simulink model "iC_3ph_MR2"  (Simulink 7.9)
settings: Solver=ode14x  StartTime=0.0  StopTime=20/60  FixedStep=Ts1  RelTol=1e-3
PostLoadFcn:
  | , if any(exist('dsrtsu_mdlpostloadfcn', 'file') == [2, 3, 6]), try dsrtsu_mdlpostloadfcn('Execute', bdroot); catch fprintf('Error in PostLoadFcn (dsrtsu_mdlpostloadfcn) for model "%s":\n %s\n', bdroot, lasterr); end, end,
InitFcn:
  | iC_ini
values from neighbouring files (symbols this model uses):
  C = Cideal+deltaC    (= 4e-05)    [IMC_calculo_limites_thetas.m]    (also in IMC_ini.m; JORGE_controlador_LCL_malha_interna.m; LCL_PAPM.m; R_in_LCL.m)
  excitacao_persistente = 0    [iC_ini.m]    (also in vC_ini.m)
  flag_time = 60/60    (= 1)    [iC_ini.m]    (also in vC_ini.m = 0)
  init_time = 60/60    (= 1)    [iC_ini.m]    (also in vC_ini.m)
  L1 = L1ideal+deltaL1    (= 0.002)    [IMC_calculo_limites_thetas.m]    (also in IMC_ini.m; LCL_PAPM.m; R_in_LCL.m; calculo_FTs.m)
  L2 = L2ideal+deltaL2+Lgideal+deltaLg    (= 0.002)    [IMC_calculo_limites_thetas.m]    (also in IMC_ini.m; LCL_PAPM.m; R_in_LCL.m; calculo_FTs.m)
  param_change_time = 60/60    (= 1)    [iC_ini.m]    (also in vC_ini.m)
  R1 = R1ideal+deltaR1    (= 1)    [IMC_calculo_limites_thetas.m]    (also in IMC_ini.m; R_in_LCL.m = 0; gera_resultados.m = 0; iC_ini.m = 0)
  R2 = R2ideal+deltaR2+Rgideal+deltaRg    (= 1)    [IMC_calculo_limites_thetas.m]    (also in IMC_ini.m; R_in_LCL.m = 0; gera_resultados.m = 0; iC_ini.m = 0)
  R_init = 10    [iC_ini.m]    (also in vC_ini.m)
  ref_phaseInv_time = 60/60    (= 1)    [iC_ini.m]    (also in vC_ini.m)
  ref_step_time = 60/60    (= 1)    [iC_ini.m]    (also in vC_ini.m)
  short_OFF_time = 61/60    (= 1.01666666667)    [iC_ini.m]    (also in vC_ini.m)
  short_ON_time = 60/60    (= 1)    [iC_ini.m]    (also in vC_ini.m)
  Ts = 0.5    [IMC_calculo_limites_thetas.m]    (also in IMC_datta_ini.m; IMC_ini.m = 8.33333333333e-05; JORGE_controlador_LCL_malha_interna.m = 8.33333333333e-05; LCL_PAPM.m = 8.33333333333e-05)
  Ts1 = Ts/10    (= 8.33333333333e-06)    [iC_ini.m]    (also in vC_ini.m)
  VCC = 1700    [iC_ini.m]    (also in vC_ini.m = 1200)
undefined symbols (not defined in the file or in its folder): D1, Delta
libraries: powerlib x38, powerlib_extras x1
(part 2 of 3)

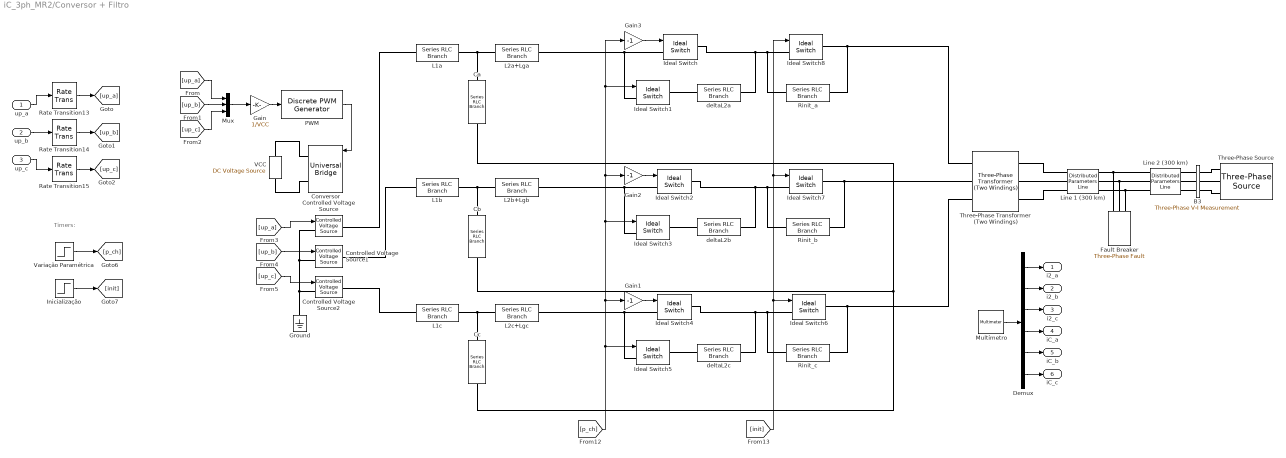
== system iC_3ph_MR2/Conversor + Filtro ==
  note: Timers:
  up_a : Inport
  up_b : Inport  Port=2
  up_c : Inport  Port=3
  B3 : powerlib/Measurements/Three-Phase V-I Measurement  VoltageMeasurement=no  SetLabelV=on  LabelV=Vabc_B3  Vpu=on  VpuLL=off  CurrentMeasurement=no  SetLabelI=on  LabelI=Iabc_B3  Ipu=on  Pbase=100e6  Vbase=735e3  OutputType=Complex  PhasorSimulation=off  PSBequivalent=0
  Ca : powerlib/Elements/Series RLC Branch  LConnTagsString=__new0  RConnTagsString=__new0  BranchType=C  Resistance=1  Inductance=1e-3  SetiL0=off  InitialCurrent=0  Capacitance=C  Setx0=off  InitialVoltage=0  Measurements=Branch current
  Cb : powerlib/Elements/Series RLC Branch  LConnTagsString=__new0  RConnTagsString=__new0  BranchType=C  Resistance=1  Inductance=1e-3  SetiL0=off  InitialCurrent=0  Capacitance=C  Setx0=off  InitialVoltage=0  Measurements=Branch current
  Cc : powerlib/Elements/Series RLC Branch  LConnTagsString=__new0  RConnTagsString=__new0  BranchType=C  Resistance=1  Inductance=1e-3  SetiL0=off  InitialCurrent=0  Capacitance=C  Setx0=off  InitialVoltage=0  Measurements=Branch current
  Controlled Voltage Source : powerlib/Electrical Sources/Controlled Voltage Source  Initialize=on  Source_Type=AC  Amplitude=0  Phase=0  Frequency=0  Measurements=None
  Controlled Voltage Source1 : powerlib/Electrical Sources/Controlled Voltage Source  Initialize=on  Source_Type=AC  Amplitude=0  Phase=0  Frequency=0  Measurements=None
  Controlled Voltage Source2 : powerlib/Electrical Sources/Controlled Voltage Source  Initialize=on  Source_Type=AC  Amplitude=0  Phase=0  Frequency=0  Measurements=None
  Conversor : powerlib/Power Electronics/Universal Bridge  Arms=3  SnubberResistance=1e5  SnubberCapacitance=inf  Device=IGBT / Diodes  Ron=1e-3  Lon=0  ForwardVoltages="[  0  0  ]"  ForwardVoltage=0  GTOparameters=[ 10e-6 , 20e-6 ]  IGBTparameters=[ 1e-6 , 2e-6 ]  Measurements=UAB UBC UCA UDC voltages  Measurements_2=None  converterType=Rectifier
  Demux : Demux  Outputs=6
  Fault Breaker : powerlib/Elements/Three-Phase Fault  FaultA=on  FaultB=off  FaultC=off  FaultResistance=0.001  GroundFault=on  GroundResistance=1  External=off  SwitchStatus=[1 0]  SwitchTimes=[ short_ON_time short_OFF_time ]  InitialStates=[0 0 1]  SnubberResistance=inf  SnubberCapacitance=inf  Measurements=Fault currents
  Gain : Gain  Gain=1/VCC  SampleTime=Ts1
  Gain1 : Gain  Gain=-1  SampleTime=Ts1
  Gain2 : Gain  Gain=-1  SampleTime=Ts1
  Gain3 : Gain  Gain=-1  SampleTime=Ts1
  Ground : powerlib/Elements/Ground  LConnTagsString=a
  Ideal Switch : powerlib/Power Electronics/Ideal Switch  Ron=0.001  Lon=0  IC=1  Rs=1e5  Cs=inf  Measurements=off
  Ideal Switch{1,3,5..8} (6 alike) : powerlib/Power Electronics/Ideal Switch  Ron=0.001  Lon=0  IC=0  Rs=1e5  Cs=inf  Measurements=off
  Ideal Switch2 : powerlib/Power Electronics/Ideal Switch  Ron=0.001  Lon=0  IC=1  Rs=1e5  Cs=inf  Measurements=off
  Ideal Switch4 : powerlib/Power Electronics/Ideal Switch  Ron=0.001  Lon=0  IC=1  Rs=1e5  Cs=inf  Measurements=off
  Inicialização : Step  Time=init_time  SampleTime=Ts1
  L1a : powerlib/Elements/Series RLC Branch  LConnTagsString=__new0  RConnTagsString=__new0  BranchType=RL  Resistance=R1  Inductance=L1  SetiL0=off  InitialCurrent=0  Capacitance=1e-6  Setx0=off  InitialVoltage=0  Measurements=Branch current
  L1b : powerlib/Elements/Series RLC Branch  LConnTagsString=__new0  RConnTagsString=__new0  BranchType=RL  Resistance=R1  Inductance=L1  SetiL0=off  InitialCurrent=0  Capacitance=1e-6  Setx0=off  InitialVoltage=0  Measurements=None
  L1c : powerlib/Elements/Series RLC Branch  LConnTagsString=__new0  RConnTagsString=__new0  BranchType=RL  Resistance=R1  Inductance=L1  SetiL0=off  InitialCurrent=0  Capacitance=1e-6  Setx0=off  InitialVoltage=0  Measurements=None
  L2a+Lga : powerlib/Elements/Series RLC Branch  LConnTagsString=__new0  RConnTagsString=__new0  BranchType=RL  Resistance=R2  Inductance=L2  SetiL0=off  InitialCurrent=0  Capacitance=1e-6  Setx0=off  InitialVoltage=0  Measurements=Branch current
  L2b+Lgb : powerlib/Elements/Series RLC Branch  LConnTagsString=__new0  RConnTagsString=__new0  BranchType=RL  Resistance=R2  Inductance=L2  SetiL0=off  InitialCurrent=0  Capacitance=1e-6  Setx0=off  InitialVoltage=0  Measurements=Branch current
  L2c+Lgc : powerlib/Elements/Series RLC Branch  LConnTagsString=__new0  RConnTagsString=__new0  BranchType=RL  Resistance=R2  Inductance=L2  SetiL0=off  InitialCurrent=0  Capacitance=1e-6  Setx0=off  InitialVoltage=0  Measurements=Branch current
  Line 1 (300 km) : powerlib/Elements/Distributed Parameters Line  Phases=3  Frequency=60  Resistance=[0.01273 0.3864]  Inductance="[0.9337e-3  4.1264e-3]"  Capacitance=[12.74e-9 7.751e-9]  Length=300  x1=[-0.0017 -2.07986760325051e-10 -7396.02996094136 -52768.9690973412;-0.00169166666666667 -2.08294895140375e-10 -7230.21513006747 -52791.9439683011;-0.00168333333333333 -2.08600974169177e-10 -7064.32893988922 -52814.3978040869;-0.001675 -2.08904994390579e-10 -6898.37302763631 -52836.3303830884;-0.00166666666666667 -2.09206952804025e-10 -6732.3490312266 -52857.74148884;-0.00165833333333333 -2.09506846429307e-10 -6566.25858924991 -52878.6309100226;-0.00165 -2.09804672306596e-10 -6400.10334095186 -52898.9984404661;-0.00164166666666667 -2.10100427496471e-10 -6233.88492621764 -52918.8438791511;-0.00163333333333333 -2.10394109079948e-10 -6067.60498555594 -52938.1670302113;-0.001625 -2.10685714158508e-10 -5901.26516008262 -52956.9677029349;-0.00161666666666667 -2.10975239854126e-10 -5734.86709150461 -52975.2457117668;-0.00160833333333333 -2.112626833093e-10 -5568.41242210365 -52993.0008763106;-0.0016 -2.11548041687081e-10 -5401.90279472016 -53010.2330213298;-0.00159166666666667 -2.11831312171096e-10 -5235.33985273692 -53026.9419767503;-0.00158333333333333 -2.12112491965579e-10 -5068.72524006292 -53043.1275776612;-0.001575 -2.123915782954e-10 -4902.06060111712 -53058.7896643173;-0.00156666666666667 -2.12668568406089e-10 -4735.34758081225 -53073.9280821402;-0.00155833333333333 -2.12943459563866e-10 -4568.58782453848 -53088.5426817197;-0.00155 -2.13216249055666e-10 -4401.7829781473 -53102.6333188156;-0.00154166666666667 -2.13486934189166e-10 -4234.9346879352 -53116.1998543591;-0.00153333333333333 -2.13755512292814e-10 -4068.04460062744 -53129.2421544539;-0.001525 -2.14021980715852e-10 -3901.11436336179 -53141.7600903777;-0.00151666666666667 -2.14286336828345e-10 -3734.14562367234 -53153.7535385837;-0.00150833333333333 -2.14548578021204e-10 -3567.14002947312 -53165.2223807013;-0.0015 -2.14808701706215e-10 -3400.09922904191 -53176.1665035377;-0.00149166666666667 -2.15066705316062e-10 -3233.02487100399 -53186.5857990787;-0.00148333333333333 -2.15322586304353e-10 -3065.91860431582 -53196.4801644902;-0.001475 -2.15576342145647e-10 -2898.78207824879 -53205.8495021188;-0.00146666666666667 -2.15827970335475e-10 -2731.61694237293 -53214.6937194929;-0.00145833333333333 -2.16077468390369e-10 -2564.42484654063 -53223.0127293236;-0.00145 -2.16324833847885e-10 -2397.20744087041 -53230.8064495056;-0.00144166666666667 -2.16570064266624e-10 -2229.96637573055 -53238.0748031181;-0.00143333333333333 -2.16813157226262e-10 -2062.70330172282 -53244.8177184255;-0.001425 -2.17054110327569e-10 -1895.41986966626 -53251.0351288777;-0.00141666666666667 -2.17292921192435e-10 -1728.11773058079 -53256.7269731115;-0.00140833333333333 -2.17529587463894e-10 -1560.798535671 -53261.8931949507;-0.0014 -2.17764106806145e-10 -1393.46393630977 -53266.5337434068;-0.00139166666666667 -2.17996476904577e-10 -1226.11558402205 -53270.6485726794;-0.00138333333333333 -2.1822669546579e-10 -1058.75513046853 -53274.2376421568;-0.001375 -2.18454760217621e-10 -891.384227429309 -53277.3009164164;-0.00136666666666667 -2.18680668909162e-10 -724.004526787619 -53279.8383652248;-0.00135833333333333 -2.18904419310786e-10 -556.617680513551 -53281.8499635385;-0.00135 -2.19126009214166e-10 -389.225340647688 -53283.3356915038;-0.00134166666666667 -2.19345436432301e-10 -221.829159284855 -53284.2955344572;-0.00133333333333333 -2.19562698799531e-10 -54.4307885577764 -53284.7294829255;-0.001325 -2.19777794171565e-10 112.968119379217 -53284.6375326256;-0.00131666666666667 -2.19990720425499e-10 280.365912366477 -53284.0196844652;-0.00130833333333333 -2.20201475459835e-10 447.760938255375 -53282.8759445421;-0.0013 -2.20410057194508e-10 615.151544924574 -53281.2063241446;-0.00129166666666667 -2.206164635709e-10 782.536080296377 -53279.0108397512;-0.00128333333333333 -2.20820692551862e-10 949.912892352986 -53276.2895130304;-0.001275 -2.21022742121738e-10 1117.28032915284 -53273.0423708406;-0.00126666666666667 -2.2122261028638e-10 1284.63673884692 -53269.2694452298;-0.00125833333333333 -2.21420295073169e-10 ...(+11171 chars)]  x2=[-0.0017 -1.41909241010387e-10 -6618.00740677681 -48900.0765944437;-0.00169166666666667 -1.41941661559306e-10 -6464.3508795585 -48920.6263316871;-0.00168333333333333 -1.4197268120133e-10 -6310.63055180677 -48940.6932420988;-0.001675 -1.42002299630307e-10 -6156.8479406792 -48960.2771276263;-0.00166666666666667 -1.42030516553915e-10 -6003.00456394808 -48979.3777949846;-0.00165833333333333 -1.42057331693664e-10 -5849.10193998542 -48997.9950556578;-0.00165 -1.42082744784901e-10 -5695.141587748 -49016.1287259012;-0.00164166666666667 -1.42106755576808e-10 -5541.12502676231 -49033.7786267426;-0.00163333333333333 -1.42129363832408e-10 -5387.05377710966 -49050.9445839847;-0.001625 -1.42150569328568e-10 -5232.92935941108 -49067.6264282065;-0.00161666666666667 -1.42170371855996e-10 -5078.75329481233 -49083.8239947647;-0.00160833333333333 -1.42188771219251e-10 -4924.52710496894 -49099.5371237962;-0.0016 -1.42205767236737e-10 -4770.25231203114 -49114.7656602184;-0.00159166666666667 -1.42221359740712e-10 -4615.93043862884 -49129.5094537321;-0.00158333333333333 -1.42235548577283e-10 -4461.56300785664 -49143.7683588218;-0.001575 -1.42248333606413e-10 -4307.15154325876 -49157.542234758;-0.00156666666666667 -1.42259714701918e-10 -4152.69756881402 -49170.830945598;-0.00155833333333333 -1.42269691751471e-10 -3998.20260892078 -49183.6343601876;-0.00155 -1.42278264656604e-10 -3843.66818838194 -49195.9523521624;-0.00154166666666667 -1.42285433332704e-10 -3689.09583238982 -49207.7847999486;-0.00153333333333333 -1.4229119770902e-10 -3534.48706651119 -49219.1315867649;-0.001525 -1.4229555772866e-10 -3379.84341667214 -49229.9926006229;-0.00151666666666667 -1.42298513348593e-10 -3225.16640914306 -49240.367734329;-0.00150833333333333 -1.42300064539646e-10 -3070.45757052359 -49250.2568854846;-0.0015 -1.42300211286512e-10 -2915.71842772749 -49259.6599564879;-0.00149166666666667 -1.42298953587741e-10 -2760.95050796762 -49268.5768545344;-0.00148333333333333 -1.42296291455747e-10 -2606.15533874088 -49277.0074916179;-0.001475 -1.42292224916804e-10 -2451.3344478131 -49284.9517845313;-0.00146666666666667 -1.42286754011046e-10 -2296.48936320396 -49292.4096548678;-0.00145833333333333 -1.42279878792469e-10 -2141.62161317193 -49299.3810290211;-0.00145 -1.4227159932893e-10 -1986.7327261992 -49305.8658381866;-0.00144166666666667 -1.42261915702142e-10 -1831.82423097653 -49311.8640183619;-0.00143333333333333 -1.42250828007681e-10 -1676.89765638823 -49317.3755103474;-0.001425 -1.42238336354975e-10 -1521.95453149706 -49322.4002597467;-0.00141666666666667 -1.42224440867314e-10 -1366.99638552911 -49326.9382169678;-0.00140833333333333 -1.4220914168184e-10 -1212.0247478587 -49330.9893372228;-0.0014 -1.42192438949549e-10 -1057.04114799335 -49334.5535805287;-0.00139166666666667 -1.42174332835291e-10 -902.047115558609 -49337.630911708;-0.00138333333333333 -1.42154823517767e-10 -747.044180283017 -49340.2213003885;-0.001375 -1.42133911189524e-10 -592.03387198296 -49342.3247210043;-0.00136666666666667 -1.4211159605696e-10 -437.017720547588 -49343.9411527954;-0.00135833333333333 -1.42087878340316e-10 -281.997255923754 -49345.0705798083;-0.00135 -1.42062758273676e-10 -126.974008100849 -49345.7129908959;-0.00134166666666667 -1.42036236104964e-10 28.0504929042545 -49345.868379718;-0.00133333333333333 -1.42008312095944e-10 183.074717062311 -49345.536744741;-0.001325 -1.41978986522216e-10 338.09713434683 -49344.7180892378;-0.00131666666666667 -1.41948259673209e-10 493.116214749123 -49343.4124212884;-0.00130833333333333 -1.41916131852186e-10 648.130428293458 -49341.6197537792;-0.0013 -1.41882603376236e-10 803.138245052127 -49339.3401044029;-0.00129166666666667 -1.41847674576271e-10 958.138135160556 -49336.573495659;-0.00128333333333333 -1.41811345797024e-10 1113.12856883241 -49333.3199548526;-0.001275 -1.41773617397045e-10 1268.10801637467 -49329.5795140949;-0.00126666666666667 -1.41734489748699e-10 1423.07494820278 -49325.3522103026;-0.00125833333333333 -1.4169396323816e-10 ...(+11177 chars)]  x3=[-0.0017 -3.70381053816407e-13 -27.7294039862372 -193.67611553396;-0.00169166666666667 -3.70681312258177e-13 -27.1208166863507 -193.762274129979;-0.00168333333333333 -3.70977912225046e-13 -26.5119617149526 -193.846520370577;-0.001675 -3.71270850789691e-13 -25.9028450811956 -193.928853424279;-0.00166666666666667 -3.71560125060927e-13 -25.2934727968152 -194.009272478489;-0.00165833333333333 -3.71845732183734e-13 -24.6838508760696 -194.087776739504;-0.00165 -3.72127669339284e-13 -24.0739853356812 -194.16436543252;-0.00164166666666667 -3.72405933744971e-13 -23.4638821947765 -194.239037801636;-0.00163333333333333 -3.72680522654439e-13 -22.8535474748273 -194.311793109866;-0.001625 -3.72951433357606e-13 -22.2429871995909 -194.382630639146;-0.00161666666666667 -3.73218663180692e-13 -21.6322073950507 -194.451549690336;-0.00160833333333333 -3.73482209486246e-13 -21.0212140893568 -194.518549583234;-0.0016 -3.73742069673174e-13 -20.4100133127665 -194.583629656578;-0.00159166666666667 -3.73998241176761e-13 -19.7986110975845 -194.646789268054;-0.00158333333333333 -3.74250721468695e-13 -19.1870134781041 -194.708027794302;-0.001575 -3.74499508057101e-13 -18.5752264905468 -194.767344630923;-0.00156666666666667 -3.74744598486553e-13 -17.9632561730031 -194.824739192482;-0.00155833333333333 -3.74985990338108e-13 -17.351108565373 -194.88021091252;-0.00155 -3.75223681229327e-13 -16.7387897093064 -194.933759243553;-0.00154166666666667 -3.75457668814297e-13 -16.126305648143 -194.985383657079;-0.00153333333333333 -3.75687950783653e-13 -15.5136624268534 -195.035083643588;-0.001525 -3.75914524864606e-13 -14.9008660919787 -195.08285871256;-0.00151666666666667 -3.76137388820962e-13 -14.2879226915714 -195.128708392475;-0.00150833333333333 -3.76356540453143e-13 -13.6748382751354 -195.172632230814;-0.0015 -3.76571977598211e-13 -13.0616188935664 -195.214629794068;-0.00149166666666667 -3.76783698129889e-13 -12.4482705990921 -195.254700667737;-0.00148333333333333 -3.76991699958579e-13 -11.8347994452125 -195.292844456338;-0.001475 -3.77195981031389e-13 -11.2212114866404 -195.329060783407;-0.00146666666666667 -3.77396539332146e-13 -10.607512779241 -195.363349291503;-0.00145833333333333 -3.77593372881421e-13 -9.99370937997291 -195.395709642214;-0.00145 -3.77786479736546e-13 -9.3798073468279 -195.426141516155;-0.00144166666666667 -3.77975857991635e-13 -8.76581273877116 -195.454644612975;-0.00143333333333333 -3.78161505777601e-13 -8.15173161568156 -195.481218651362;-0.001425 -3.78343421262174e-13 -7.53757003829192 -195.50586336904;-0.00141666666666667 -3.78521602649923e-13 -6.92333406812905 -195.528578522775;-0.00140833333333333 -3.7869604818227e-13 -6.30902976745399 -195.549363888378;-0.0014 -3.78866756137506e-13 -5.69466319920217 -195.568219260705;-0.00139166666666667 -3.79033724830814e-13 -5.08024042692358 -195.585144453663;-0.00138333333333333 -3.7919695261428e-13 -4.46576751472298 -195.600139300206;-0.001375 -3.79356437876912e-13 -3.85125052719994 -195.613203652342;-0.00136666666666667 -3.79512179044655e-13 -3.23669552938895 -195.624337381129;-0.00135833333333333 -3.79664174580405e-13 -2.62210858669984 -195.633540376683;-0.00135 -3.79812422984029e-13 -2.00749576485755 -195.640812548174;-0.00134166666666667 -3.79956922792375e-13 -1.39286312984251 -195.646153823829;-0.00133333333333333 -3.80097672579287e-13 -0.778216747830726 -195.649564150931;-0.001325 -3.80234670955623e-13 -0.163562685133797 -195.651043495821;-0.00131666666666667 -3.80367916569263e-13 0.45109299186079 -195.6505918439;-0.00130833333333333 -3.80497408105128e-13 1.06574421674968 -195.648209199625;-0.0013 -3.80623144285187e-13 1.68038492317338 -195.643895586511;-0.00129166666666667 -3.80745123868477e-13 2.29500904487631 -195.637651047133;-0.00128333333333333 -3.80863345651106e-13 2.90961051576649 -195.62947564312;-0.001275 -3.80977808466275e-13 3.52418326997552 -195.619369455162;-0.00126666666666667 -3.81088511184281e-13 4.13872124191849 -195.607332583003;-0.00125833333333333 -3.81195452712534e-13 ...(+11162 chars)]  x4=[-0.0017 -8.97577288364198e-15 -97.1520132574431 -167.719905551199;-0.00169166666666667 -9.90341611680488e-15 -96.624627075456 -168.024289436398;-0.00168333333333333 -1.08309616072489e-14 -96.0962872474087 -168.327014989695;-0.001675 -1.17584002004744e-14 -95.5669989878018 -168.62807922331;-0.00166666666666667 -1.26857227430371e-14 -95.036767520497 -168.927479165861;-0.00165833333333333 -1.36129200826377e-14 -94.5055980786645 -169.225211862392;-0.00165 -1.45399830682128e-14 -93.9734959047326 -169.5212743744;-0.00164166666666667 -1.54669025500252e-14 -93.4404662503346 -169.815663779869;-0.00163333333333333 -1.63936693797535e-14 -92.9065143762582 -170.108377173294;-0.001625 -1.73202744105835e-14 -92.3716455523928 -170.399411665711;-0.00161666666666667 -1.82467084972975e-14 -91.8358650576778 -170.688764384729;-0.00160833333333333 -1.91729624963652e-14 -91.2991781800502 -170.976432474552;-0.0016 -2.00990272660334e-14 -90.761590216393 -171.262413096012;-0.00159166666666667 -2.10248936664168e-14 -90.2231064724823 -171.546703426596;-0.00158333333333333 -2.19505525595879e-14 -89.6837322629353 -171.829300660474;-0.001575 -2.2875994809667e-14 -89.1434729111575 -172.110202008525;-0.00156666666666667 -2.38012112829127e-14 -88.6023337492909 -172.389404698365;-0.00155833333333333 -2.4726192847812e-14 -88.0603201181603 -172.666905974378;-0.00155 -2.56509303751702e-14 -87.5174373672216 -172.942703097737;-0.00154166666666667 -2.65754147382014e-14 -86.9736908545083 -173.216793346436;-0.00153333333333333 -2.7499636812618e-14 -86.4290859465789 -173.489174015315;-0.001525 -2.84235874767214e-14 -85.8836280184641 -173.759842416088;-0.00151666666666667 -2.93472576114914e-14 -85.3373224536133 -174.028795877365;-0.00150833333333333 -3.02706381006767e-14 -84.7901746438421 -174.296031744685;-0.0015 -3.11937198308847e-14 -84.2421899892782 -174.561547380538;-0.00149166666666667 -3.21164936916715e-14 -83.6933738983091 -174.825340164392;-0.00148333333333333 -3.30389505756314e-14 -83.1437317875281 -175.087407492718;-0.001475 -3.39610813784875e-14 -82.5932690816807 -175.347746779018;-0.00146666666666667 -3.48828769991811e-14 -82.0419912136118 -175.606355453848;-0.00145833333333333 -3.58043283399615e-14 -81.4899036242113 -175.863230964844;-0.00145 -3.67254263064759e-14 -80.9370117623608 -176.11837077675;-0.00144166666666667 -3.76461618078593e-14 -80.3833210848798 -176.371772371439;-0.00143333333333333 -3.85665257568241e-14 -79.8288370564718 -176.623433247938;-0.001425 -3.94865090697496e-14 -79.2735651496702 -176.873350922457;-0.00141666666666667 -4.04061026667719e-14 -78.7175108447846 -177.121522928408;-0.00140833333333333 -4.13252974718735e-14 -78.1606796298466 -177.367946816436;-0.0014 -4.22440844129728e-14 -77.6030770005553 -177.612620154434;-0.00139166666666667 -4.31624544220135e-14 -77.0447084602237 -177.855540527577;-0.00138333333333333 -4.40803984350545e-14 -76.4855795197238 -178.096705538338;-0.001375 -4.49979073923588e-14 -75.9256956974325 -178.336112806516;-0.00136666666666667 -4.59149722384837e-14 -75.365062519177 -178.573759969257;-0.00135833333333333 -4.68315839223691e-14 -74.8036855181807 -178.809644681081;-0.00135 -4.77477333974279e-14 -74.2415702350077 -179.043764613901;-0.00134166666666667 -4.86634116216347e-14 -73.6787222175091 -179.276117457046;-0.00133333333333333 -4.95786095576149e-14 -73.1151470207675 -179.506700917289;-0.001325 -5.04933181727345e-14 -72.5508502070426 -179.735512718863;-0.00131666666666667 -5.14075284391886e-14 -71.9858373457161 -179.96255060349;-0.00130833333333333 -5.23212313340912e-14 -71.4201140132368 -180.187812330395;-0.0013 -5.32344178395634e-14 -70.8536857930657 -180.411295676338;-0.00129166666666667 -5.41470789428232e-14 -70.2865582756206 -180.632998435627;-0.00128333333333333 -5.50592056362739e-14 -69.7187370582212 -180.852918420146;-0.001275 -5.59707889175932e-14 -69.1502277450336 -181.071053459374;-0.00126666666666667 -5.68818197898223e-14 -68.5810359470152 -181.287401400405;-0.00125833333333333 ...(+11312 chars)]  x5=0.00169662470098723  Measurements=None
      settings: AttributesFormatString=\n
  Line 2 (300 km) : powerlib/Elements/Distributed Parameters Line  Phases=3  Frequency=60  Resistance=[0.01273 0.3864]  Inductance="[0.9337e-3  4.1264e-3]"  Capacitance=[12.74e-9 7.751e-9]  Length=300  x1=[-0.0017 -1.41909241010387e-10 -6618.00740677681 -48900.0765944437;-0.00169166666666667 -1.41941661559306e-10 -6464.3508795585 -48920.6263316871;-0.00168333333333333 -1.4197268120133e-10 -6310.63055180677 -48940.6932420988;-0.001675 -1.42002299630307e-10 -6156.8479406792 -48960.2771276263;-0.00166666666666667 -1.42030516553915e-10 -6003.00456394808 -48979.3777949846;-0.00165833333333333 -1.42057331693664e-10 -5849.10193998542 -48997.9950556578;-0.00165 -1.42082744784901e-10 -5695.141587748 -49016.1287259012;-0.00164166666666667 -1.42106755576808e-10 -5541.12502676231 -49033.7786267426;-0.00163333333333333 -1.42129363832408e-10 -5387.05377710966 -49050.9445839847;-0.001625 -1.42150569328568e-10 -5232.92935941108 -49067.6264282065;-0.00161666666666667 -1.42170371855996e-10 -5078.75329481233 -49083.8239947647;-0.00160833333333333 -1.42188771219251e-10 -4924.52710496894 -49099.5371237962;-0.0016 -1.42205767236737e-10 -4770.25231203114 -49114.7656602184;-0.00159166666666667 -1.42221359740712e-10 -4615.93043862884 -49129.5094537321;-0.00158333333333333 -1.42235548577283e-10 -4461.56300785664 -49143.7683588218;-0.001575 -1.42248333606413e-10 -4307.15154325876 -49157.542234758;-0.00156666666666667 -1.42259714701918e-10 -4152.69756881402 -49170.830945598;-0.00155833333333333 -1.42269691751471e-10 -3998.20260892078 -49183.6343601876;-0.00155 -1.42278264656604e-10 -3843.66818838194 -49195.9523521624;-0.00154166666666667 -1.42285433332704e-10 -3689.09583238982 -49207.7847999486;-0.00153333333333333 -1.4229119770902e-10 -3534.48706651119 -49219.1315867649;-0.001525 -1.4229555772866e-10 -3379.84341667214 -49229.9926006229;-0.00151666666666667 -1.42298513348593e-10 -3225.16640914306 -49240.367734329;-0.00150833333333333 -1.42300064539646e-10 -3070.45757052359 -49250.2568854846;-0.0015 -1.42300211286512e-10 -2915.71842772749 -49259.6599564879;-0.00149166666666667 -1.42298953587741e-10 -2760.95050796762 -49268.5768545344;-0.00148333333333333 -1.42296291455747e-10 -2606.15533874088 -49277.0074916179;-0.001475 -1.42292224916804e-10 -2451.3344478131 -49284.9517845313;-0.00146666666666667 -1.42286754011046e-10 -2296.48936320396 -49292.4096548678;-0.00145833333333333 -1.42279878792469e-10 -2141.62161317193 -49299.3810290211;-0.00145 -1.4227159932893e-10 -1986.7327261992 -49305.8658381866;-0.00144166666666667 -1.42261915702142e-10 -1831.82423097653 -49311.8640183619;-0.00143333333333333 -1.42250828007681e-10 -1676.89765638823 -49317.3755103474;-0.001425 -1.42238336354975e-10 -1521.95453149706 -49322.4002597467;-0.00141666666666667 -1.42224440867314e-10 -1366.99638552911 -49326.9382169678;-0.00140833333333333 -1.4220914168184e-10 -1212.0247478587 -49330.9893372228;-0.0014 -1.42192438949549e-10 -1057.04114799335 -49334.5535805287;-0.00139166666666667 -1.42174332835291e-10 -902.047115558609 -49337.630911708;-0.00138333333333333 -1.42154823517767e-10 -747.044180283017 -49340.2213003885;-0.001375 -1.42133911189524e-10 -592.03387198296 -49342.3247210043;-0.00136666666666667 -1.4211159605696e-10 -437.017720547588 -49343.9411527954;-0.00135833333333333 -1.42087878340316e-10 -281.997255923754 -49345.0705798083;-0.00135 -1.42062758273676e-10 -126.974008100849 -49345.7129908959;-0.00134166666666667 -1.42036236104964e-10 28.0504929042545 -49345.868379718;-0.00133333333333333 -1.42008312095944e-10 183.074717062311 -49345.536744741;-0.001325 -1.41978986522216e-10 338.09713434683 -49344.7180892378;-0.00131666666666667 -1.41948259673209e-10 493.116214749123 -49343.4124212884;-0.00130833333333333 -1.41916131852186e-10 648.130428293458 -49341.6197537792;-0.0013 -1.41882603376236e-10 803.138245052127 -49339.3401044029;-0.00129166666666667 -1.41847674576271e-10 958.138135160556 -49336.573495659;-0.00128333333333333 -1.41811345797024e-10 1113.12856883241 -49333.3199548526;-0.001275 -1.41773617397045e-10 1268.10801637467 -49329.5795140949;-0.00126666666666667 -1.41734489748699e-10 1423.07494820278 -49325.3522103026;-0.00125833333333333 -1.4169396323816e-10 ...(+11177 chars)]  x2=[-0.0017 -1.56442071045307e-11 -4583.41557044112 -37720.1439036556;-0.00169166666666667 -1.56451442295778e-11 -4464.89182015718 -37734.3569633582;-0.00168333333333333 -1.56459269433674e-11 -4346.32400319353 -37748.1976001916;-0.001675 -1.56465552381747e-11 -4227.71328976664 -37761.6656775542;-0.00166666666666667 -1.56470291077985e-11 -4109.06085051639 -37774.7610625216;-0.00165833333333333 -1.5647348547562e-11 -3990.36785649442 -37787.4836258476;-0.00165 -1.56475135543124e-11 -3871.6354791527 -37799.8332419657;-0.00164166666666667 -1.56475241264212e-11 -3752.86489033184 -37811.80978899;-0.00163333333333333 -1.5647380263784e-11 -3634.0572622496 -37823.413148717;-0.001625 -1.56470819678208e-11 -3515.21376748931 -37834.6432066261;-0.00161666666666667 -1.56466292414755e-11 -3396.33557898829 -37845.4998518813;-0.00160833333333333 -1.56460220892163e-11 -3277.42387002626 -37855.9829773317;-0.0016 -1.56452605170357e-11 -3158.47981421378 -37866.0924795133;-0.00159166666666667 -1.56443445324501e-11 -3039.50458548066 -37875.8282586492;-0.00158333333333333 -1.56432741444998e-11 -2920.49935806439 -37885.1902186513;-0.001575 -1.56420493637491e-11 -2801.4653064985 -37894.1782671208;-0.00156666666666667 -1.56406702022862e-11 -2682.40360560104 -37902.7923153494;-0.00155833333333333 -1.56391366737227e-11 -2563.31543046291 -37911.0322783197;-0.00155 -1.56374487931941e-11 -2444.20195643635 -37918.8980747068;-0.00154166666666667 -1.5635606577359e-11 -2325.06435912323 -37926.3896268783;-0.00153333333333333 -1.56336100443993e-11 -2205.90381436356 -37933.5068608957;-0.001525 -1.563145921402e-11 -2086.7214982238 -37940.2497065148;-0.00151666666666667 -1.56291541074489e-11 -1967.51858698529 -37946.6180971864;-0.00150833333333333 -1.56266947474366e-11 -1848.29625713266 -37952.611970057;-0.0015 -1.56240811582558e-11 -1729.05568534215 -37958.2312659696;-0.00149166666666667 -1.56213133657017e-11 -1609.79804847007 -37963.475929464;-0.00148333333333333 -1.56183913970913e-11 -1490.52452354116 -37968.3459087774;-0.001475 -1.56153152812632e-11 -1371.23628773695 -37972.8411558451;-0.00146666666666667 -1.56120850485774e-11 -1251.93451838417 -37976.9616263008;-0.00145833333333333 -1.5608700730915e-11 -1132.62039294312 -37980.7072794773;-0.00145 -1.56051623616779e-11 -1013.29508899604 -37984.0780784063;-0.00144166666666667 -1.56014699757883e-11 -893.959784235531 -37987.0739898194;-0.00143333333333333 -1.55976236096887e-11 -774.61565645285 -37989.6949841483;-0.001425 -1.55936233013411e-11 -655.263883526366 -37991.9410355248;-0.00141666666666667 -1.55894690902268e-11 -535.905643409893 -37993.8121217812;-0.00140833333333333 -1.55851610173464e-11 -416.542114121075 -37995.3082244507;-0.0014 -1.55806991252187e-11 -297.174473729752 -37996.4293287673;-0.00139166666666667 -1.55760834578808e-11 -177.803900346345 -37997.1754236663;-0.00138333333333333 -1.55713140608875e-11 -58.4315721102266 -37997.5465017839;-0.001375 -1.55663909813109e-11 60.9413328219107 -37997.5425594577;-0.00136666666666667 -1.55613142677396e-11 180.313636287709 -37997.1635967267;-0.00135833333333333 -1.55560839702789e-11 299.684160130704 -37996.4096173311;-0.00135 -1.55507001405496e-11 419.05172621203 -37995.2806287124;-0.00134166666666667 -1.55451628316881e-11 538.415156421997 -37993.7766420131;-0.00133333333333333 -1.55394720983452e-11 657.773272691731 -37991.8976720771;-0.001325 -1.55336279966862e-11 777.124897004822 -37989.6437374491;-0.00131666666666667 -1.55276305843901e-11 896.468851408921 -37987.0148603743;-0.00130833333333333 -1.55214799206489e-11 1015.80395802737 -37984.0110667989;-0.0013 -1.55151760661671e-11 1135.12903907085 -37980.632386369;-0.00129166666666667 -1.55087190831613e-11 1254.44291684899 -37976.8788524309;-0.00128333333333333 -1.55021090353593e-11 1373.74441378198 -37972.7505020304;-0.001275 -1.54953459879996e-11 1493.0323524122 -37968.2473759126;-0.00126666666666667 -1.54884300078306e-11 1612.30555541587 -37963.3695185217;-0.00125833333333333 -1.54813611631105e-11 ...(+11172 chars)]  x3=[-0.0017 -1.28062535702143e-13 48.7742194936725 -189.74083377891;-0.00169166666666667 -1.27384616282729e-13 49.370066231705 -189.586668968601;-0.00168333333333333 -1.26705439628579e-13 49.9654257071152 -189.430633014409;-0.001675 -1.26025012442893e-13 50.5602920439456 -189.272727456345;-0.00166666666666667 -1.25343341441213e-13 51.1546593711055 -189.112953852873;-0.00165833333333333 -1.24660433351356e-13 51.7485218224295 -188.951313780895;-0.00165 -1.23976294913349e-13 52.3418735367347 -188.787808835733;-0.00164166666666667 -1.23290932879363e-13 52.9347086578794 -188.622440631114;-0.00163333333333333 -1.22604354013644e-13 53.5270213348202 -188.455210799156;-0.001625 -1.21916565092448e-13 54.1188057216702 -188.286120990351;-0.00161666666666667 -1.21227572903974e-13 54.7100559777564 -188.115172873545;-0.00160833333333333 -1.20537384248297e-13 55.3007662676775 -187.942368135928;-0.0016 -1.198460059373e-13 55.8909307613612 -187.767708483012;-0.00159166666666667 -1.19153444794609e-13 56.4805436341225 -187.591195638619;-0.00158333333333333 -1.18459707655522e-13 57.0695990667202 -187.412831344859;-0.001575 -1.17764801366944e-13 57.6580912454151 -187.232617362115;-0.00156666666666667 -1.17068732787321e-13 58.2460143620268 -187.050555469027;-0.00155833333333333 -1.16371508786567e-13 58.8333626139917 -186.866647462471;-0.00155 -1.15673136246003e-13 59.4201302044196 -186.680895157546;-0.00154166666666667 -1.14973622058283e-13 60.0063113421512 -186.493300387552;-0.00153333333333333 -1.1427297312733e-13 60.5919002418154 -186.303865003973;-0.001525 -1.13571196368267e-13 61.1768911238862 -186.112590876461;-0.00151666666666667 -1.12868298707345e-13 61.7612782147396 -185.919479892814;-0.00150833333333333 -1.12164287081883e-13 62.3450557467112 -185.724533958958;-0.0015 -1.11459168440189e-13 62.9282179581522 -185.527754998933;-0.00149166666666667 -1.107529497415e-13 63.5107590934872 -185.329144954866;-0.00148333333333333 -1.10045637955911e-13 64.0926734032702 -185.128705786959;-0.001475 -1.09337240064302e-13 64.6739551442419 -184.926439473466;-0.00146666666666667 -1.08627763058275e-13 65.2545985793864 -184.722348010672;-0.00145833333333333 -1.07917213940081e-13 65.8345979779872 -184.51643341288;-0.00145 -1.07205599722554e-13 66.4139476156844 -184.308697712381;-0.00144166666666667 -1.06492927429038e-13 66.9926417745311 -184.099142959445;-0.00143333333333333 -1.05779204093321e-13 67.5706747430496 -183.887771222292;-0.001425 -1.05064436759565e-13 68.1480408162876 -183.674584587075;-0.00141666666666667 -1.04348632482234e-13 68.7247342958753 -183.45958515786;-0.00140833333333333 -1.03631798326027e-13 69.3007494900808 -183.242775056606;-0.0014 -1.02913941365809e-13 69.8760807138667 -183.02415642314;-0.00139166666666667 -1.02195068686538e-13 70.4507222889461 -182.80373141514;-0.00138333333333333 -1.01475187383197e-13 71.0246685438385 -182.581502208112;-0.001375 -1.00754304560723e-13 71.5979138139262 -182.357470995368;-0.00136666666666667 -1.0003242733394e-13 72.1704524415099 -182.131639988006;-0.00135833333333333 -9.93095628274832e-14 72.7422787758643 -181.904011414887;-0.00135 -9.85857181757344e-14 73.3133871732945 -181.674587522613;-0.00134166666666667 -9.7860900522748e-14 73.8837719971911 -181.443370575505;-0.00133333333333333 -9.71351170221814e-14 74.4534276180862 -181.210362855581;-0.001325 -9.64083748372249e-14 75.0223484137087 -180.975566662533;-0.00131666666666667 -9.56806811405303e-14 75.5905287690401 -180.738984313705;-0.00130833333333333 -9.49520431141407e-14 76.1579630763697 -180.500618144069;-0.0013 -9.42224679494193e-14 76.72464573535 -180.260470506204;-0.00129166666666667 -9.34919628469784e-14 77.2905711530518 -180.018543770268;-0.00128333333333333 -9.27605350166084e-14 77.8557337440199 -179.774840323982;-0.001275 -9.20281916772068e-14 78.4201279303275 -179.5293625726;-0.00126666666666667 -9.12949400567065e-14 78.9837481416319 -179.282112938888;-0.00125833333333333 -9.05607873920052e-14 79.5465888152292 -179.0330938631;-0.00125 ...(+11100 chars)]  x4=[-0.0017 -6.38107087677307e-14 -152.47288977289 -118.697101129343;-0.00169166666666667 -6.47829879288146e-14 -152.099240022438 -119.175522305555;-0.00168333333333333 -6.57546277079616e-14 -151.724089113893 -119.652767267475;-0.001675 -6.67256185154795e-14 -151.347440749842 -120.128831304888;-0.00166666666666667 -6.76959507680807e-14 -150.969298647652 -120.603709719235;-0.00165833333333333 -6.86656148889778e-14 -150.589666539432 -121.077397823655;-0.00165 -6.96346013079774e-14 -150.208548172 -121.549890943041;-0.00164166666666667 -7.06029004615748e-14 -149.825947306839 -122.021184414074;-0.00163333333333333 -7.15705027930481e-14 -149.441867720065 -122.491273585279;-0.001625 -7.2537398752553e-14 -149.056313202389 -122.960153817066;-0.00161666666666667 -7.35035787972168e-14 -148.669287559078 -123.427820481775;-0.00160833333333333 -7.44690333912324e-14 -148.280794609919 -123.894268963726;-0.0016 -7.54337530059529e-14 -147.890838189181 -124.359494659261;-0.00159166666666667 -7.6397728119985e-14 -147.499422145576 -124.823492976789;-0.00158333333333333 -7.73609492192836e-14 -147.106550342222 -125.286259336835;-0.001575 -7.83234067972452e-14 -146.712226656605 -125.747789172081;-0.00156666666666667 -7.92850913548022e-14 -146.316454980542 -126.208077927414;-0.00155833333333333 -8.02459934005163e-14 -145.919239220138 -126.667121059971;-0.00155 -8.1206103450672e-14 -145.520583295753 -127.124914039181;-0.00154166666666667 -8.21654120293709e-14 -145.12049114196 -127.581452346811;-0.00153333333333333 -8.31239096686247e-14 -144.718966707507 -128.036731477013;-0.001525 -8.40815869084485e-14 -144.316013955278 -128.490746936366;-0.00151666666666667 -8.50384342969546e-14 -143.911636862254 -128.943494243921;-0.00150833333333333 -8.59944423904456e-14 -143.505839419473 -129.394968931244;-0.0015 -8.69496017535076e-14 -143.098625631993 -129.845166542463;-0.00149166666666667 -8.79039029591032e-14 -142.68999951885 -130.294082634308;-0.00148333333333333 -8.88573365886649e-14 -142.279965113017 -130.74171277616;-0.001475 -8.98098932321875e-14 -141.86852646137 -131.188052550089;-0.00146666666666667 -9.07615634883218e-14 -141.455687624641 -131.633097550902;-0.00145833333333333 -9.17123379644664e-14 -141.041452677383 -132.076843386185;-0.00145 -9.26622072768609e-14 -140.625825707927 -132.519285676345;-0.00144166666666667 -9.36111620506789e-14 -140.208810818346 -132.960420054656;-0.00143333333333333 -9.45591929201198e-14 -139.790412124406 -133.400242167299;-0.001425 -9.55062905285017e-14 -139.370633755533 -133.838747673408;-0.00141666666666667 -9.64524455283535e-14 -138.949479854772 -134.27593224511;-0.00140833333333333 -9.73976485815074e-14 -138.526954578741 -134.71179156757;-0.0014 -9.83418903591908e-14 -138.103062097594 -135.146321339033;-0.00139166666666667 -9.92851615421186e-14 -137.677806594979 -135.579517270865;-0.00138333333333333 -1.00227452820585e-13 -137.251192267995 -136.011375087598;-0.001375 -1.01168754894555e-13 -136.823223327154 -136.441890526968;-0.00136666666666667 -1.02109058473759e-13 -136.393903996336 -136.871059339962;-0.00135833333333333 -1.03048354277778e-13 -135.963238512751 -137.298877290858;-0.00135 -1.03986633036143e-13 -135.531231126892 -137.725340157265;-0.00134166666666667 -1.0492388548842e-13 -135.097886102498 -138.150443730166;-0.00133333333333333 -1.05860102384308e-13 -134.663207716509 -138.574183813962;-0.001325 -1.06795274483722e-13 -134.227200259026 -138.996556226507;-0.00131666666666667 -1.07729392556892e-13 -133.789868033266 -139.417556799158;-0.00130833333333333 -1.0866244738445e-13 -133.351215355521 -139.837181376809;-0.0013 -1.09594429757521e-13 -132.911246555118 -140.255425817934;-0.00129166666666667 -1.10525330477816e-13 -132.469965974369 -140.672285994629;-0.00128333333333333 -1.11455140357719e-13 -132.027377968536 -141.087757792654;-0.001275 -1.12383850220383e-13 -131.583486905784 -141.501837111468;-0.00126666666666667 -1.13311450899817e-13 -131.138297167139 -141.914519864277;-0.00125833333333333 ...(+11342 chars)]  x5=0.00169662470098723  Measurements=None
      settings: AttributesFormatString=\n
  Multímetro : powerlib/Measurements/Multimeter  PhasorSimulation=off  OutputType=Complex  sel=[9 10 11 5 6 7]  L=14  Gain=[1 1 1 1 1 1]  yselected={'Ib: Conversor + Filtro/L2a+Lga','Ib: Conversor + Filtro/L2b+Lgb','Ib: Conversor + Filtro/L2c+Lgc','Ib: Conversor + Filtro/Ca','Ib: Conversor + Filtro/Cb','Ib: Conversor + Filtro/Cc'};  PSBOutputType=1  PSBequivalent=0  AxesSetting=[0,0.1,-100,100]  Display=0  SavedBlockNames=-11
  Mux : Mux  Inputs=3
  PWM : powerlib_extras/Discrete  Control Blocks/Discrete PWM Generator  GeneratorMode="3-arm  bridge (6 pulses)"  Fc=12000  Ts=Ts1  Internal=off  mIndex=0.4  Freq=60  Phase=0
  Rate Transition13 : RateTransition  OutPortSampleTime=Ts1
  Rate Transition14 : RateTransition  OutPortSampleTime=Ts1
  Rate Transition15 : RateTransition  OutPortSampleTime=Ts1
  Rinit_a : powerlib/Elements/Series RLC Branch  LConnTagsString=__new0  RConnTagsString=__new0  BranchType=RL  Resistance=R_init  Inductance=5*L2  SetiL0=off  InitialCurrent=0  Capacitance=1e-6  Setx0=off  InitialVoltage=0  Measurements=None
  Rinit_b : powerlib/Elements/Series RLC Branch  LConnTagsString=__new0  RConnTagsString=__new0  BranchType=RL  Resistance=R_init  Inductance=5*L2  SetiL0=off  InitialCurrent=0  Capacitance=1e-6  Setx0=off  InitialVoltage=0  Measurements=None
  Rinit_c : powerlib/Elements/Series RLC Branch  LConnTagsString=__new0  RConnTagsString=__new0  BranchType=RL  Resistance=R_init  Inductance=5*L2  SetiL0=off  InitialCurrent=0  Capacitance=1e-6  Setx0=off  InitialVoltage=0  Measurements=None
  Three-Phase Transformer (Two Windings) : powerlib/Elements/Three-Phase Transformer (Two Windings)  Winding1Connection=Yg  UNITS=pu  NominalPower=[ 2.5e6 , 60 ]  Winding1=[ 440 , 0.002 , 0.08 ]  Winding2Connection=Delta (D1)  Winding2=[ 34.5e3 , 0.002 , 0.08 ]  SetSaturation=off  Rm=500  Lm=500  Saturation=[ 0,0 ; 0.0024,1.2 ; 1.0,1.52 ]  Hysteresis=off  DataFile='hysteresis'  SetInitialFlux=off  InitialFluxes=[ 0.8 , -0.8 , 0.7 ]  Measurements=None  MoreParameters=off  BreakLoop=off  DataType=off  TransfoNumber=1
  Three-Phase Source : powerlib/Electrical Sources/Three-Phase Source  Voltage=38e3  PhaseAngle=0  Frequency=60  InternalConnection=Yg  SpecifyImpedance=off  Resistance=1  Inductance=0.01e-3  ShortCircuitLevel=100e6  BaseVoltage=380e3  XRratio=7  BusType=swing  Pref=0  Qref=0  Qmin=-inf  Qmax=inf
  VCC : powerlib/Electrical Sources/DC Voltage Source  Amplitude=VCC  Measurements=None
  Variação Paramétrica : Step  Time=param_change_time  Before=-1  SampleTime=Ts1
  deltaL2a : powerlib/Elements/Series RLC Branch  LConnTagsString=__new0  RConnTagsString=__new0  BranchType=RL  Resistance=0  Inductance=5*L2  SetiL0=off  InitialCurrent=0  Capacitance=1e-6  Setx0=off  InitialVoltage=0  Measurements=None
  deltaL2b : powerlib/Elements/Series RLC Branch  LConnTagsString=__new0  RConnTagsString=__new0  BranchType=RL  Resistance=0  Inductance=5*L2  SetiL0=off  InitialCurrent=0  Capacitance=1e-6  Setx0=off  InitialVoltage=0  Measurements=None
  deltaL2c : powerlib/Elements/Series RLC Branch  LConnTagsString=__new0  RConnTagsString=__new0  BranchType=RL  Resistance=0  Inductance=5*L2  SetiL0=off  InitialCurrent=0  Capacitance=1e-6  Setx0=off  InitialVoltage=0  Measurements=None
  i2_a : Outport
  i2_b : Outport  Port=2
  i2_c : Outport  Port=3
  iC_a : Outport  Port=4
  iC_b : Outport  Port=5
  iC_c : Outport  Port=6
  wires:
  Gain/1 -> PWM/1
  up_a/1 -> Rate Transition13/1
  up_b/1 -> Rate Transition14/1
  up_c/1 -> Rate Transition15/1
  Rate Transition13/1 -> [up_a]
  Rate Transition14/1 -> [up_b]
  Rate Transition15/1 -> [up_c]
  PWM/1 -> Conversor/1
  Mux/1 -> Gain/1
  [up_a] -> Controlled Voltage Source/1
  [up_b] -> Controlled Voltage Source1/1
  [up_c] -> Controlled Voltage Source2/1
  Multímetro/1 -> Demux/1
  Demux/1 -> i2_a/1
  Demux/2 -> i2_b/1
  Demux/3 -> i2_c/1
  Demux/4 -> iC_a/1
  Demux/5 -> iC_b/1
  Demux/6 -> iC_c/1
  [up_b] -> Mux/2
  [up_a] -> Mux/1
  [up_c] -> Mux/3
  Variação Paramétrica/1 -> [p_ch]
  Gain1/1 -> Ideal Switch4/1
  Gain2/1 -> Ideal Switch2/1
  Gain3/1 -> Ideal Switch/1
  [init] -> Ideal Switch6/1, Ideal Switch8/1, Ideal Switch7/1
  Inicialização/1 -> [init]
  [p_ch] -> Gain1/1, Gain2/1, Gain3/1, Ideal Switch1/1, Ideal Switch3/1, Ideal Switch5/1
  connections:
  Ideal Switch/RConn1 -- deltaL2a/RConn1 -- Ideal Switch8/LConn1 -- Rinit_a/LConn1
  Ca/LConn1 -- L2a+Lga/LConn1 -- L1a/RConn1
  Cb/LConn1 -- L1b/RConn1 -- L2b+Lgb/LConn1
  Cc/LConn1 -- L1c/RConn1 -- L2c+Lgc/LConn1
  Conversor/RConn1 -- VCC/RConn1
  VCC/LConn1 -- Conversor/RConn2
  L2a+Lga/RConn1 -- Ideal Switch/LConn1 -- Ideal Switch1/LConn1
  deltaL2a/LConn1 -- Ideal Switch1/RConn1
  L2b+Lgb/RConn1 -- Ideal Switch2/LConn1 -- Ideal Switch3/LConn1
  deltaL2b/LConn1 -- Ideal Switch3/RConn1
  L2c+Lgc/RConn1 -- Ideal Switch4/LConn1 -- Ideal Switch5/LConn1
  deltaL2c/LConn1 -- Ideal Switch5/RConn1
  Cc/RConn1 -- Cb/RConn1 -- Ca/RConn1
  Rinit_a/RConn1 -- Ideal Switch8/RConn1 -- Three-Phase Transformer (Two Windings)/LConn1
  Rinit_b/RConn1 -- Ideal Switch7/RConn1 -- Three-Phase Transformer (Two Windings)/LConn2
  Rinit_c/RConn1 -- Ideal Switch6/RConn1 -- Three-Phase Transformer (Two Windings)/LConn3
  Ideal Switch4/RConn1 -- deltaL2c/RConn1 -- Ideal Switch6/LConn1 -- Rinit_c/LConn1
  Ideal Switch2/RConn1 -- deltaL2b/RConn1 -- Ideal Switch7/LConn1 -- Rinit_b/LConn1
  Controlled Voltage Source2/LConn1 -- Controlled Voltage Source1/LConn1 -- Controlled Voltage Source/LConn1 -- Ground/LConn1
  Line 2 (300 km)/LConn2 -- Fault Breaker/LConn2 -- Line 1 (300 km)/RConn2
  Line 2 (300 km)/LConn1 -- Fault Breaker/LConn1 -- Line 1 (300 km)/RConn1
  Line 1 (300 km)/RConn3 -- Fault Breaker/LConn3 -- Line 2 (300 km)/LConn3
  B3/RConn1 -- Three-Phase Source/RConn1
  B3/RConn2 -- Three-Phase Source/RConn2
  B3/RConn3 -- Three-Phase Source/RConn3
  Line 2 (300 km)/RConn3 -- B3/LConn3
  B3/LConn2 -- Line 2 (300 km)/RConn2
  Line 2 (300 km)/RConn1 -- B3/LConn1
  Three-Phase Transformer (Two Windings)/RConn2 -- Line 1 (300 km)/LConn2
  Line 1 (300 km)/LConn1 -- Three-Phase Transformer (Two Windings)/RConn1
  Line 1 (300 km)/LConn3 -- Three-Phase Transformer (Two Windings)/RConn3
  Controlled Voltage Source/RConn1 -- L1a/LConn1
  L1b/LConn1 -- Controlled Voltage Source1/RConn1
  L1c/LConn1 -- Controlled Voltage Source2/RConn1
